simulink model "prototype_phaseshifted"  (R2015b)
settings: Solver=VariableStepAuto  StartTime=0.0  StopTime=10.0  RelTol=1e-3
libraries: simulink x3, powerlib_meascontrol x3
settings Model: Creator=hakan  LastModifiedBy=hakan

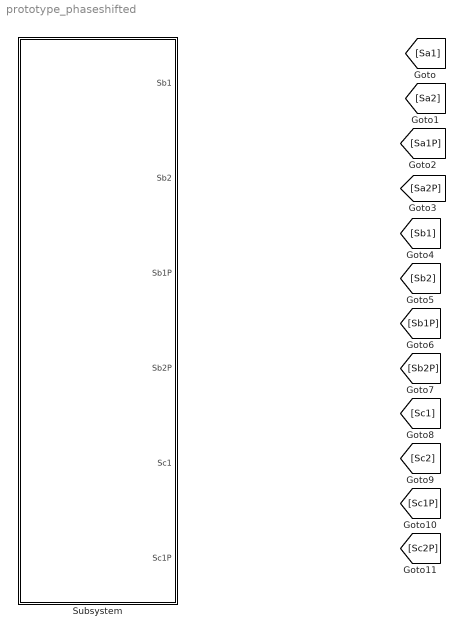
== system prototype_phaseshifted ==
  Subsystem : Subsystem
  wires:
  ? -> [Sa1]
  ? -> [Sa2]
  ? -> [Sa1P]
  ? -> [Sa2P]
  ? -> [Sb1]
  ? -> [Sb2]
  ? -> [Sb1P]
  ? -> [Sb2P]
  ? -> [Sc1]
  ? -> [Sc2]
  ? -> [Sc1P]
  ? -> [Sc2P]

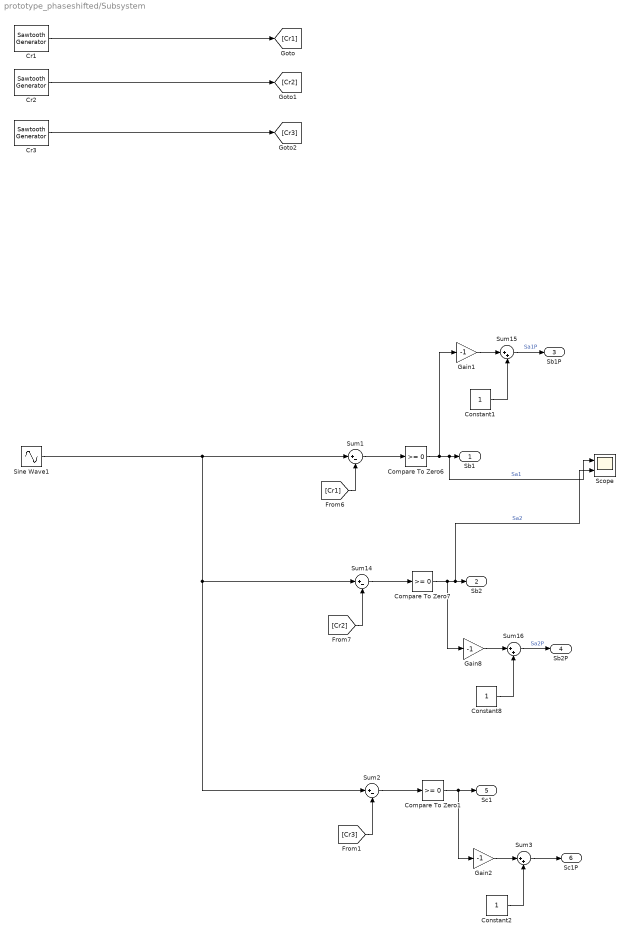
== system prototype_phaseshifted/Subsystem ==
  Compare To Zero1 : simulink/Logic and Bit Operations/Compare To Zero  relop=>=  OutDataTypeStr=boolean
  Compare To Zero6 : simulink/Logic and Bit Operations/Compare To Zero  relop=>=  OutDataTypeStr=boolean
  Compare To Zero7 : simulink/Logic and Bit Operations/Compare To Zero  relop=>=  OutDataTypeStr=boolean
  Constant1 : Constant
  Constant2 : Constant
  Constant8 : Constant
  "Cr1 " : powerlib_meascontrol/Pulse & Signal Generators/Sawtooth Generator  Freq=2000  Phase=0  Ts=0
  "Cr2 " : powerlib_meascontrol/Pulse & Signal Generators/Sawtooth Generator  Freq=2000  Phase=120  Ts=0
  Cr3 : powerlib_meascontrol/Pulse & Signal Generators/Sawtooth Generator  Freq=2000  Phase=-120  Ts=0
  Gain1 : Gain  Gain=-1
  Gain2 : Gain  Gain=-1
  Gain8 : Gain  Gain=-1
  Scope : Scope  NumInputPorts=2
  Sine Wave1 : Sin  Amplitude=0.8  Frequency=100*pi  SampleTime=0
  Sum1 : Sum  Inputs=|+-
  Sum14 : Sum  Inputs=|+-
  Sum15 : Sum  Inputs=|++
  Sum16 : Sum  Inputs=|++
  Sum2 : Sum  Inputs=|+-
  Sum3 : Sum  Inputs=|++
  Sb1 : Outport
  Sb2 : Outport  Port=2
  Sb1P : Outport  Port=3
  Sb2P : Outport  Port=4
  Sc1 : Outport  Port=5
  "Sc1P " : Outport  Port=6
  wires:
  "Cr1 "/1 -> [Cr1]
  "Cr2 "/1 -> [Cr2]
  Compare To Zero6/1 -> Scope/1, Sb1/1, Gain1/1  "Sa1"
  Compare To Zero7/1 -> Scope/2, Sb2/1, Gain8/1  "Sa2"
  Constant1/1 -> Sum15/2
  Gain1/1 -> Sum15/1
  Sum15/1 -> Sb1P/1  "Sa1P"
  Constant8/1 -> Sum16/2
  Gain8/1 -> Sum16/1
  [Cr1] -> Sum1/2
  [Cr2] -> Sum14/2
  Sum1/1 -> Compare To Zero6/1
  Sum14/1 -> Compare To Zero7/1
  Sine Wave1/1 -> Sum2/1, Sum14/1, Sum1/1
  Sum16/1 -> Sb2P/1  "Sa2P"
  Cr3/1 -> [Cr3]
  Compare To Zero1/1 -> Gain2/1, Sc1/1
  Constant2/1 -> Sum3/2
  Gain2/1 -> Sum3/1
  [Cr3] -> Sum2/2
  Sum3/1 -> "Sc1P "/1
  Sum2/1 -> Compare To Zero1/1
